simulink model "BaseEngineController_LS"  (Simulink 7.7)
settings: Solver=FixedStepDiscrete  StartTime=0.0  StopTime=10.0  RelTol=1e-3
PreLoadFcn:
  | try, eval([bdroot '_setup']); catch, eval('model_setup', ''); end
InitFcn:
  | try, eval([bdroot '_setup']); catch, eval('model_setup', ''); end
undefined symbols (not defined in the file): ECU555, High, motohawk_build_version, motohawk_trunc_name, motohawk_vardec_config_group, motohawk_vardec_path, True
libraries: MotoHawk_lib x1418, motohawk_control_primitives_lib x183, motohawk_engine_lib x32, simulink x21, motohawk_annotations_lib x9, AutoDoc_lib x8, simulink_extras x4, motohawk_ccp_examples_lib x1, motohawk_control_primitives_motoshare_lib x1
(part 13 of 27)

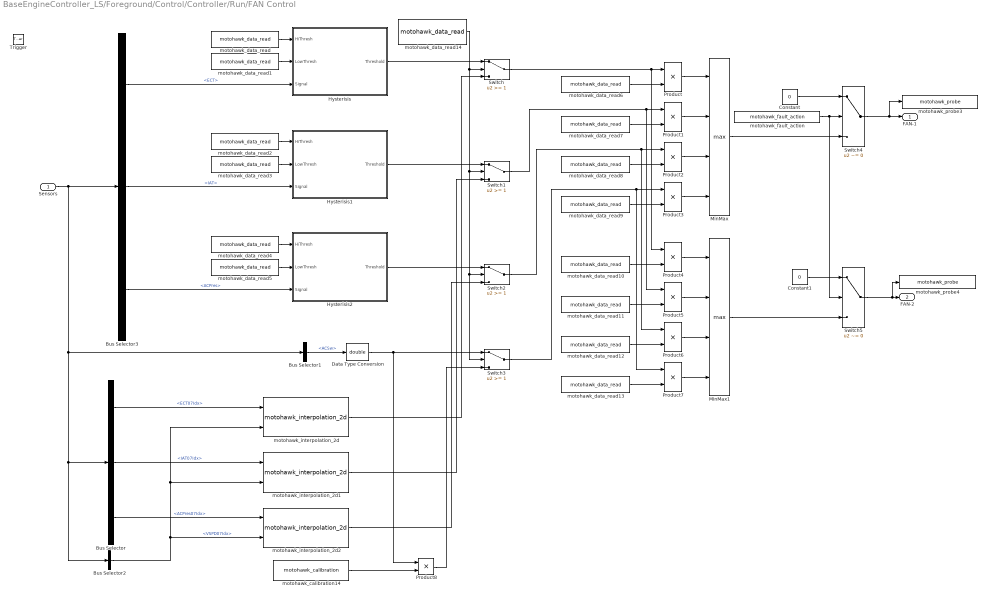
== system BaseEngineController_LS/Foreground/Control/Controller/Run/FAN Control ==
  Sensors : Inport
  Trigger : TriggerPort  TriggerType=function-call
  Bus Selector : BusSelector  OutputSignals=RawIndexes.ECT07Idx,RawIndexes.IAT07Idx,RawIndexes.ACPres07Idx
  Bus Selector1 : BusSelector  OutputSignals=Raw.Digital.ACSw
  Bus Selector2 : BusSelector  OutputSignals=RawIndexes.VSPD07Idx
  Bus Selector3 : BusSelector  OutputSignals=Raw.NonLinearSensors.ECT,Raw.NonLinearSensors.IAT,Raw.LinearSensors.ACPres
  Constant : Constant  Value=0
  Constant1 : Constant  Value=0
  Data Type Conversion : DataTypeConversion  OutDataTypeStr=double
  Hysterisis : Subsystem  AncestorBlock=motohawk_control_primitives_lib/Hysterisis
      mask Display:
      | patch([0 0 1 1], [0 0.075 0.075 0], [230/255 0/255 0/255])
      | patch([0 0 1 1], [0.025 0.05 0.05 0.025], [150/255 0/255 0/255])
      | patch([0 0 1 1], [0 0.025 0.025 0], [0/255 0/255 0/255])
      | 
      | disp('HYSTERISIS')
  Hysterisis1 : Subsystem  AncestorBlock=motohawk_control_primitives_lib/Hysterisis
      mask Display:
      | patch([0 0 1 1], [0 0.075 0.075 0], [230/255 0/255 0/255])
      | patch([0 0 1 1], [0.025 0.05 0.05 0.025], [150/255 0/255 0/255])
      | patch([0 0 1 1], [0 0.025 0.025 0], [0/255 0/255 0/255])
      | 
      | disp('HYSTERISIS')
  Hysterisis2 : Subsystem  AncestorBlock=motohawk_control_primitives_lib/Hysterisis
      mask Display:
      | patch([0 0 1 1], [0 0.075 0.075 0], [230/255 0/255 0/255])
      | patch([0 0 1 1], [0.025 0.05 0.05 0.025], [150/255 0/255 0/255])
      | patch([0 0 1 1], [0 0.025 0.025 0], [0/255 0/255 0/255])
      | 
      | disp('HYSTERISIS')
  MinMax : MinMax  Function=max  Inputs=4
  MinMax1 : MinMax  Function=max  Inputs=4
  Product{,1..8} (9 alike) : Product  RndMeth=Zero
  Switch{,1..3} (4 alike) : Switch  Threshold=1
  Switch4 : Switch  Criteria=u2 ~= 0
  Switch5 : Switch  Criteria=u2 ~= 0
  motohawk_calibration14 : MotoHawk_lib/Calibration & Probing Blocks/motohawk_calibration  nam='ACSwFanSpeed'  val=50  storage=Calibration  show_more=on  name_source=Use Parameter  data_type=uint8  read_level=1  write_level=1  ovr_cals=on  view_as=Number  enum_struct={'Disabled', 'Enabled'}  vector_style=Wide Row  use_help_units=on  help='Fan speed % req for AC Sw 0 to disable'  units='%'  use_header_enum=off  row_header_enum={}  col_header_enum={}  use_min_max=on  min_val=0  max_val=100  use_precision=off  precision=''  gain=1  offset=0  exp=1  use_mototune_group=off  mototune_group=motohawk_vardec_path(gcb)
  motohawk_data_read : MotoHawk_lib/Data Storage Blocks/motohawk_data_read  source=Lookup By Name  structure=Scalar  operation=Read scalar from location by index  sz_vec=4  sz_row=2  sz_col=3  typ=double  nam='ECTFanOn'  checkNull=on  struct_inst_name='MyData'  struct_nam='MyStruct'
  motohawk_data_read1 : MotoHawk_lib/Data Storage Blocks/motohawk_data_read  source=Lookup By Name  structure=Scalar  operation=Read scalar from location by index  sz_vec=4  sz_row=2  sz_col=3  typ=double  nam='ECTFanOff'  checkNull=on  struct_inst_name='MyData'  struct_nam='MyStruct'
  motohawk_data_read10 : MotoHawk_lib/Data Storage Blocks/motohawk_data_read  source=Lookup By Name  structure=Scalar  operation=Read scalar from location by index  sz_vec=4  sz_row=2  sz_col=3  typ=boolean  nam='Fan2ECT'  checkNull=on  struct_inst_name='MyData'  struct_nam='MyStruct'
  motohawk_data_read11 : MotoHawk_lib/Data Storage Blocks/motohawk_data_read  source=Lookup By Name  structure=Scalar  operation=Read scalar from location by index  sz_vec=4  sz_row=2  sz_col=3  typ=boolean  nam='Fan2IAT'  checkNull=on  struct_inst_name='MyData'  struct_nam='MyStruct'
  motohawk_data_read12 : MotoHawk_lib/Data Storage Blocks/motohawk_data_read  source=Lookup By Name  structure=Scalar  operation=Read scalar from location by index  sz_vec=4  sz_row=2  sz_col=3  typ=boolean  nam='Fan2ACPres'  checkNull=on  struct_inst_name='MyData'  struct_nam='MyStruct'
  motohawk_data_read13 : MotoHawk_lib/Data Storage Blocks/motohawk_data_read  source=Lookup By Name  structure=Scalar  operation=Read scalar from location by index  sz_vec=4  sz_row=2  sz_col=3  typ=boolean  nam='Fan2ACSw'  checkNull=on  struct_inst_name='MyData'  struct_nam='MyStruct'
  motohawk_data_read14 : MotoHawk_lib/Data Storage Blocks/motohawk_data_read  source=Lookup By Name  structure=Scalar  operation=Read scalar from location by index  sz_vec=4  sz_row=2  sz_col=3  typ=boolean  nam='FAN_Mode'  checkNull=on  struct_inst_name='MyData'  struct_nam='MyStruct'
  motohawk_data_read2 : MotoHawk_lib/Data Storage Blocks/motohawk_data_read  source=Lookup By Name  structure=Scalar  operation=Read scalar from location by index  sz_vec=4  sz_row=2  sz_col=3  typ=double  nam='IATFanOn'  checkNull=on  struct_inst_name='MyData'  struct_nam='MyStruct'
  motohawk_data_read3 : MotoHawk_lib/Data Storage Blocks/motohawk_data_read  source=Lookup By Name  structure=Scalar  operation=Read scalar from location by index  sz_vec=4  sz_row=2  sz_col=3  typ=double  nam='IATFanOff'  checkNull=on  struct_inst_name='MyData'  struct_nam='MyStruct'
  motohawk_data_read4 : MotoHawk_lib/Data Storage Blocks/motohawk_data_read  source=Lookup By Name  structure=Scalar  operation=Read scalar from location by index  sz_vec=4  sz_row=2  sz_col=3  typ=double  nam='ACPresFanOn'  checkNull=on  struct_inst_name='MyData'  struct_nam='MyStruct'
  motohawk_data_read5 : MotoHawk_lib/Data Storage Blocks/motohawk_data_read  source=Lookup By Name  structure=Scalar  operation=Read scalar from location by index  sz_vec=4  sz_row=2  sz_col=3  typ=double  nam='ACPresFanOff'  checkNull=on  struct_inst_name='MyData'  struct_nam='MyStruct'
  motohawk_data_read6 : MotoHawk_lib/Data Storage Blocks/motohawk_data_read  source=Lookup By Name  structure=Scalar  operation=Read scalar from location by index  sz_vec=4  sz_row=2  sz_col=3  typ=boolean  nam='Fan1ECT'  checkNull=on  struct_inst_name='MyData'  struct_nam='MyStruct'
  motohawk_data_read7 : MotoHawk_lib/Data Storage Blocks/motohawk_data_read  source=Lookup By Name  structure=Scalar  operation=Read scalar from location by index  sz_vec=4  sz_row=2  sz_col=3  typ=boolean  nam='Fan1IAT'  checkNull=on  struct_inst_name='MyData'  struct_nam='MyStruct'
  motohawk_data_read8 : MotoHawk_lib/Data Storage Blocks/motohawk_data_read  source=Lookup By Name  structure=Scalar  operation=Read scalar from location by index  sz_vec=4  sz_row=2  sz_col=3  typ=boolean  nam='Fan1ACPres'  checkNull=on  struct_inst_name='MyData'  struct_nam='MyStruct'
  motohawk_data_read9 : MotoHawk_lib/Data Storage Blocks/motohawk_data_read  source=Lookup By Name  structure=Scalar  operation=Read scalar from location by index  sz_vec=4  sz_row=2  sz_col=3  typ=boolean  nam='Fan1ACSw'  checkNull=on  struct_inst_name='MyData'  struct_nam='MyStruct'
  motohawk_fault_action : MotoHawk_lib/Fault Management Blocks/motohawk_fault_action  nam='DisableFanRun'  output_status=on  eval_nam=DisableFanRun
  motohawk_interpolation_2d : MotoHawk_lib/Lookup Tables/motohawk_interpolation_2d  nam='ECTFanSpeed'  table_data=ones(7)  show_more=off  data_type=Inherit from 'Table Data'  storage=NonAdaptive  read_level=1  write_level=1  ovr_cals=on  use_help=off  help=''  units=''  use_min_max=off  min_val=-inf  max_val=inf  use_precision=off  precision=''  gain=1  offset=0  exp=1  use_links=off  row_prelookup_block=''  col_prelookup_block=''  output_name=''  use_mototune_group=off  mototune_group=motohawk_vardec_path(gcb)
  motohawk_interpolation_2d1 : MotoHawk_lib/Lookup Tables/motohawk_interpolation_2d  nam='IATFanSpeed'  table_data=ones(7)  show_more=off  data_type=Inherit from 'Table Data'  storage=NonAdaptive  read_level=1  write_level=1  ovr_cals=on  use_help=off  help=''  units=''  use_min_max=off  min_val=-inf  max_val=inf  use_precision=off  precision=''  gain=1  offset=0  exp=1  use_links=off  row_prelookup_block=''  col_prelookup_block=''  output_name=''  use_mototune_group=off  mototune_group=motohawk_vardec_path(gcb)
  motohawk_interpolation_2d2 : MotoHawk_lib/Lookup Tables/motohawk_interpolation_2d  nam='ACPresFanSpeed'  table_data=ones(7)  show_more=off  data_type=Inherit from 'Table Data'  storage=NonAdaptive  read_level=1  write_level=1  ovr_cals=on  use_help=off  help=''  units=''  use_min_max=off  min_val=-inf  max_val=inf  use_precision=off  precision=''  gain=1  offset=0  exp=1  use_links=off  row_prelookup_block=''  col_prelookup_block=''  output_name=''  use_mototune_group=off  mototune_group=motohawk_vardec_path(gcb)
  motohawk_probe3 : MotoHawk_lib/Calibration & Probing Blocks/motohawk_probe  nam='Fan1Cmd'  show_more=on  name_source=Use Parameter  read_level=1  view_as=Number  enum_struct={'Disabled', 'Enabled'}  vector_style=Wide Row  use_help_units=on  help='FAN 1 final request'  units='%'  use_header_enum=off  row_header_enum={}  col_header_enum={}  use_precision=off  precision=''  gain=1  offset=0  exp=1  use_mototune_group=off  mototune_group=motohawk_vardec_path(gcb)
  motohawk_probe4 : MotoHawk_lib/Calibration & Probing Blocks/motohawk_probe  nam='Fan2Cmd'  show_more=on  name_source=Use Parameter  read_level=1  view_as=Number  enum_struct={'Disabled', 'Enabled'}  vector_style=Wide Row  use_help_units=on  help='Fan 2 final command'  units='%'  use_header_enum=off  row_header_enum={}  col_header_enum={}  use_precision=off  precision=''  gain=1  offset=0  exp=1  use_mototune_group=off  mototune_group=motohawk_vardec_path(gcb)
  FAN-1 : Outport
  FAN-2 : Outport  Port=2
  wires:
  Sensors/1 -> Bus Selector1/1, Bus Selector2/1, Bus Selector/1, Bus Selector3/1
  motohawk_data_read1/1 -> Hysterisis/2(LowThresh)
  motohawk_data_read/1 -> Hysterisis/1(HiThresh)
  motohawk_data_read2/1 -> Hysterisis1/1(HiThresh)
  motohawk_data_read3/1 -> Hysterisis1/2(LowThresh)
  motohawk_data_read4/1 -> Hysterisis2/1(HiThresh)
  Product/1 -> MinMax/1
  motohawk_data_read6/1 -> Product/2
  Product1/1 -> MinMax/2
  motohawk_data_read7/1 -> Product1/2
  Product2/1 -> MinMax/3
  motohawk_data_read8/1 -> Product2/2
  Product3/1 -> MinMax/4
  motohawk_data_read9/1 -> Product3/2
  Bus Selector1/1 -> Data Type Conversion/1  "<ACSw>"
  Product4/1 -> MinMax1/1
  motohawk_data_read10/1 -> Product4/2
  Product5/1 -> MinMax1/2
  motohawk_data_read11/1 -> Product5/2
  Product6/1 -> MinMax1/3
  motohawk_data_read12/1 -> Product6/2
  Product7/1 -> MinMax1/4
  motohawk_data_read5/1 -> Hysterisis2/2(LowThresh)
  motohawk_data_read13/1 -> Product7/2
  Data Type Conversion/1 -> Product8/1, Switch3/1
  motohawk_calibration14/1 -> Product8/2
  Hysterisis/1(Threshold) -> Switch/1
  motohawk_data_read14/1 -> Switch/2, Switch1/2, Switch2/2, Switch3/2
  Hysterisis1/1(Threshold) -> Switch1/1
  Hysterisis2/1(Threshold) -> Switch2/1
  Product8/1 -> Switch3/3
  motohawk_interpolation_2d2/1 -> Switch2/3
  motohawk_interpolation_2d1/1 -> Switch1/3
  motohawk_interpolation_2d/1 -> Switch/3
  Switch/1 -> Product/1, Product4/1
  Switch1/1 -> Product1/1, Product5/1
  Switch2/1 -> Product2/1, Product6/1
  Switch3/1 -> Product3/1, Product7/1
  Switch4/1 -> FAN-1/1, motohawk_probe3/1
  MinMax/1 -> Switch4/3
  motohawk_fault_action/1 -> Switch4/2, Switch5/2
  Constant/1 -> Switch4/1
  MinMax1/1 -> Switch5/3
  Switch5/1 -> FAN-2/1, motohawk_probe4/1
  Constant1/1 -> Switch5/1
  Bus Selector/1 -> motohawk_interpolation_2d/1  "<ECT07Idx>"
  Bus Selector/2 -> motohawk_interpolation_2d1/1  "<IAT07Idx>"
  Bus Selector/3 -> motohawk_interpolation_2d2/1  "<ACPres07Idx>"
  Bus Selector2/1 -> motohawk_interpolation_2d2/2, motohawk_interpolation_2d1/2, motohawk_interpolation_2d/2  "<VSPD07Idx>"
  Bus Selector3/1 -> Hysterisis/3(Signal)  "<ECT>"
  Bus Selector3/2 -> Hysterisis1/3(Signal)  "<IAT>"
  Bus Selector3/3 -> Hysterisis2/3(Signal)  "<ACPres>"

== system BaseEngineController_LS/Foreground/Control/Controller/Run/Fuel System Manager ==
  Sensors : Inport
  O2_Info : Inport  Port=2
  Bus Selector : BusSelector  OutputSignals=O2Error.O2Cals
  DesiredFuelCalc : Subsystem
  Fuel Calculation : Subsystem
      mask Display:
      | patch([0 0 1 1], 0.5*[0 0.075 0.075 0], [230/255 0/255 0/255])
      | patch([0 0 1 1], 0.5*[0.025 0.05 0.05 0.025], [150/255 0/255 0/255])
      | patch([0 0 1 1], 0.5*[0 0.025 0.025 0], [0/255 0/255 0/255])
      | 
      | disp('BASE FUEL');
  Injector Manager : Subsystem  TreatAsAtomicUnit=on
      mask Display:
      | patch([0 0 1 1], 0.5*[0 0.075 0.075 0], [230/255 0/255 0/255])
      | patch([0 0 1 1], 0.5*[0.025 0.05 0.05 0.025], [150/255 0/255 0/255])
      | patch([0 0 1 1], 0.5*[0 0.025 0.025 0], [0/255 0/255 0/255])
  O2 Fuel Adapt : Subsystem  TreatAsAtomicUnit=on
      mask Display:
      | patch([0 0 1 1], 0.5*[0 0.075 0.075 0], [230/255 0/255 0/255])
      | patch([0 0 1 1], 0.5*[0.025 0.05 0.05 0.025], [150/255 0/255 0/255])
      | patch([0 0 1 1], 0.5*[0 0.025 0.025 0], [0/255 0/255 0/255])
  DesiredFuel : Outport
  InjTiming : Outport  Port=2
  EOI : Outport  Port=3
  wires:
  O2_Info/1 -> Fuel Calculation/2(O2Info), O2 Fuel Adapt/1(O2 Info), Bus Selector/1
  Fuel Calculation/1(Fuel) -> Injector Manager/1(Fuel)
  Injector Manager/1(PrimaryInjTiming) -> InjTiming/1
  Injector Manager/2(MakeUpInjTiming) -> EOI/1
  Sensors/1 -> O2 Fuel Adapt/2(Sensors), Injector Manager/2(Sensors), Fuel Calculation/1(Sensors)
  DesiredFuelCalc/1(DesiredFuel) -> DesiredFuel/1
  Bus Selector/1 -> DesiredFuelCalc/2(BankCals)  "<O2Cals>"
  Injector Manager/3(FPC) -> DesiredFuelCalc/1(FPC)
  O2 Fuel Adapt/1("Adapt Fuel Mult Bank A ") -> DesiredFuelCalc/3(BankAMult)
  O2 Fuel Adapt/2(Adapt Fuel Mult Bank B) -> DesiredFuelCalc/4(BankBMult)

== system BaseEngineController_LS/Foreground/Control/Controller/Run/IAC Characterization ==
  MinGovINFO : Inport
  Bus Selector4 : BusSelector  OutputSignals=OnIdle,BaseAirOfst,MinGovAirPID
  Constant : Constant  Value=0
  Constant1 : Constant  Value=100
  Constant2 : Constant  Value=0
  Logical Operator : Logic  Operator=NOT  AllPortsSameDT=off  OutDataTypeStr=boolean
  Sum : Sum  Inputs=|+-
  Sum2 : Sum
  Switch1 : Switch  Criteria=u2 > Threshold
  Switch4 : Switch  Threshold=1
  motohawk_data_read : MotoHawk_lib/Data Storage Blocks/motohawk_data_read  source=Lookup By Name  structure=Scalar  operation=Read scalar from location by index  sz_vec=4  sz_row=2  sz_col=3  typ=uint8  nam='IACType'  checkNull=on  struct_inst_name='MyData'  struct_nam='MyStruct'
  IAC-P : Outport
  IAC-S : Outport  Port=2
  wires:
  motohawk_data_read/1 -> Switch1/2
  Switch1/1 -> IAC-S/1
  Constant/1 -> Switch1/3
  Constant1/1 -> Sum/1
  Sum/1 -> Switch1/1
  Logical Operator/1 -> Switch4/2
  Bus Selector4/1 -> Logical Operator/1  "<OnIdle>"
  Bus Selector4/3 -> Sum2/2  "<MinGovAirPID>"
  Bus Selector4/2 -> Sum2/1  "<BaseAirOfst>"
  MinGovINFO/1 -> Bus Selector4/1
  Switch4/1 -> Sum/2, IAC-P/1
  Constant2/1 -> Switch4/1
  Sum2/1 -> Switch4/3

== system BaseEngineController_LS/Foreground/Control/Controller/Run/MaxGovernor ==
  MinGovInfo : Inport
  Sensors : Inport  Port=2
  Trigger : TriggerPort  TriggerType=function-call
  Bus Creator : BusCreator  Inputs=2
  Bus Selector1 : BusSelector  OutputSignals=BaseAirOfst
  Bus Selector2 : BusSelector  OutputSignals=RawProcessed.ETCRequest
  Bus Selector3 : BusSelector  OutputSignals=VirtualIndexes.RPMAccel17Idx
  Bus Selector4 : BusSelector  OutputSignals=Raw.RPMInst
  Bus Selector5 : BusSelector  OutputSignals=Raw.RPMInst,Raw.Digital.ClutchSw
  Data Type Conversion : DataTypeConversion  OutDataTypeStr=double
  Data Type Conversion1 : DataTypeConversion  OutDataTypeStr=double
  I-Term Preload : Subsystem  TreatAsAtomicUnit=on
  MaxGovState : Subsystem
  Ramp RPM : Subsystem
      mask Display: disp('RAMP RPM\nINTO STEADY-STATE');
  Sum : Sum  Inputs=|++
  Terminator : Terminator
  Trigger Pre-load : Subsystem
  Unit Delay : UnitDelay  SampleTime=-1
  Universal PID (Tunable & Scheduled) : Subsystem  AncestorBlock=motohawk_control_primitives_lib/Universal PID (Tunable & Scheduled)  mask(Universal PID (Tunable)){nam='MaxGov', prefix='MaxGov', samp_time=-1, units='%', group=motohawk_vardec_path(gcb)}
      mask prompts: nam "Name"; samp_time "Sample Time"; group "MotoTune Group String"
      mask help:
      | This block wraps a 'Universal PID' block to provide gain scheduling and calibrations and probes for most parameters.
      |
      | If 'Sample Time' is -1, then extra code and RAM will be generated to dynamically calculate dt.
      mask init:
      | grp = [group ' | ' nam];
      mask Display:
      | patch([0 0 1 1], [0 0.075 0.075 0], [230/255 0/255 0/255])
      | patch([0 0 1 1], [0.025 0.05 0.05 0.025], [150/255 0/255 0/255])
      | patch([0 0 1 1], [0 0.025 0.025 0], [0/255 0/255 0/255])
      | 
      | disp([nam '\n(PID w/ Gain Schedules)']);
  motohawk_probe : MotoHawk_lib/Calibration & Probing Blocks/motohawk_probe  nam='TPSRequestLookupAirOfst'  show_more=on  name_source=Use Parameter  read_level=1  view_as=Number  enum_struct={'Disabled', 'Enabled'}  vector_style=Wide Row  use_help_units=on  help=''  units=''  use_header_enum=off  row_header_enum={}  col_header_enum={}  use_precision=on  precision=''  gain=1  offset=0  exp=1  use_mototune_group=on  mototune_group=motohawk_vardec_path(gcb)
  motohawk_probe2 : MotoHawk_lib/Calibration & Probing Blocks/motohawk_probe  nam='MaxGovOutput'  show_more=on  name_source=Use Parameter  read_level=1  view_as=Number  enum_struct={'Disabled', 'Enabled'}  vector_style=Wide Row  use_help_units=on  help=''  units=''  use_header_enum=off  row_header_enum={}  col_header_enum={}  use_precision=on  precision=''  gain=1  offset=0  exp=1  use_mototune_group=on  mototune_group=motohawk_vardec_path(gcb)
  MaxGovInfo : Outport
  wires:
  MinGovInfo/1 -> Bus Selector1/1
  Bus Creator/1 -> MaxGovInfo/1
  Bus Selector1/1 -> Sum/1  "<BaseAirOfst>"
  Bus Selector2/1 -> Sum/2  "<ETCRequest>"
  Sensors/1 -> Bus Selector2/1, Bus Selector5/1, Bus Selector3/1, Bus Selector4/1, MaxGovState/3(Sensors)
  Sum/1 -> I-Term Preload/1(TotalETCReq), MaxGovState/2(TotalETCReq), motohawk_probe/1
  Bus Selector3/1 -> I-Term Preload/2(RPMAccelIdx)  "<RPMAccel17Idx>"
  I-Term Preload/1(ITerm Preload) -> Universal PID (Tunable & Scheduled)/1(ITerm IC)
  MaxGovState/1(ETCMode) -> Bus Creator/1, Unit Delay/1  "MaxGovState"
  Trigger Pre-load/1(Trigger) -> MaxGovState/1(RPMEntryCriteria)
  Bus Selector4/1 -> Data Type Conversion1/1  "<RPMInst>"
  Bus Selector5/1 -> Trigger Pre-load/1(RPM)  "<RPMInst>"
  Universal PID (Tunable & Scheduled)/1(MaxGovOut) -> Bus Creator/2, motohawk_probe2/1  "MaxGovPID"
  Universal PID (Tunable & Scheduled)/2(MaxGovITerm) -> Terminator/1
  Trigger Pre-load/2(BaseRPMSetpoint) -> Data Type Conversion/1
  Unit Delay/1 -> Ramp RPM/1(OnIdle)
  MaxGovState/3(PIDHold) -> Universal PID (Tunable & Scheduled)/3(Hold PID)
  Ramp RPM/1(RPMSetPt) -> Universal PID (Tunable & Scheduled)/4(SetPoint)
  MaxGovState/2(PIDReset) -> Universal PID (Tunable & Scheduled)/2(Reset All)
  Bus Selector5/2 -> Trigger Pre-load/2(GearState)  "<ClutchSw>"
  Data Type Conversion/1 -> Ramp RPM/2(TargetRPM), MaxGovState/4(TargetRPM)
  Data Type Conversion1/1 -> Universal PID (Tunable & Scheduled)/5(Actual), Ramp RPM/3(RPM)

== system BaseEngineController_LS/Foreground/Control/Controller/Run/MinGovernor ==
  Sensors : Inport
  AC : Inport  Port=2
  Trigger : TriggerPort  TriggerType=function-call
  AiflowOffset : Subsystem  TreatAsAtomicUnit=on
  Base Airflow Table Adapt : Subsystem  TreatAsAtomicUnit=on
  Base RPM Set Pt : Subsystem  TreatAsAtomicUnit=on
  Bus Creator2 : BusCreator  Inputs=5
  Bus Selector : BusSelector  OutputSignals=Raw.RPM
  Bus Selector1 : BusSelector  OutputSignals=Raw.RPMInst
  Constant1 : Constant  Value=0  OutDataTypeStr=Inherit: Inherit via back propagation  SampleTime=-1
  Data Type Conversion : DataTypeConversion  OutDataTypeStr=double
  Data Type Conversion1 : DataTypeConversion  SaturateOnIntegerOverflow=on  RndMeth=Zero
  Handoff Alpha : motohawk_control_primitives_lib/Handoff Alpha  SystemSampleTime=-1  samp_time=-1
  Hit  Crossing1 : HitCross  HitCrossingOffset=.5  HitCrossingDirection=falling
  Idle State Determination : Subsystem
      mask Display: disp('IDLE STATE\nDETERMINATION');
  Logical Operator : Logic  Operator=OR  AllPortsSameDT=off
  MotoringDetection : Subsystem
  OnIdle State : motohawk_control_primitives_lib/CompareTo  SystemSampleTime=-1  op===  val=0
  Product : Product  SaturateOnIntegerOverflow=on  InputSameDT=on  OutDataTypeStr=Inherit: Same as first input
  Product1 : Product  SaturateOnIntegerOverflow=on  InputSameDT=on  OutDataTypeStr=Inherit: Same as first input
  Ramp RPM : Subsystem
      mask Display: disp('RAMP RPM\nINTO IDLE STATE');
  Unit Delay1 : UnitDelay  SampleTime=-1
  Unit Delay2 : UnitDelay  SampleTime=-1
  Unit Delay3 : UnitDelay  SampleTime=-1
  Universal PD (Tunable & Scheduled) : Subsystem  AncestorBlock=motohawk_control_primitives_lib/Universal PD (Tunable & Scheduled)  mask(Universal PD (Tunable)){nam='SpkMinGov', prefix='SpkMinGov', samp_time=-1, units='degCA', group=motohawk_vardec_path(gcb)}
      mask prompts: nam "Name"; samp_time "Sample Time"; group "MotoTune Group String"
      mask help:
      | This block wraps a 'Universal PD' block to provide gain scheduling and calibrations and probes for most parameters.
      |
      | If 'Sample Time' is -1, then extra code and RAM will be generated to dynamically calculate dt.
      mask init:
      | grp = [group ' | ' nam];
      mask Display:
      | patch([0 0 1 1], [0 0.075 0.075 0], [230/255 0/255 0/255])
      | patch([0 0 1 1], [0.025 0.05 0.05 0.025], [150/255 0/255 0/255])
      | patch([0 0 1 1], [0 0.025 0.025 0], [0/255 0/255 0/255])
      | 
      | disp([nam '\n(PD w/ Gain Schedules)']);
  Universal PID (Tunable & Scheduled) : Subsystem  AncestorBlock=motohawk_control_primitives_lib/Universal PID (Tunable & Scheduled)  mask(Universal PID (Tunable)){nam='AirMinGov', prefix='AirMinGov', samp_time=-1, units='%', group=motohawk_vardec_path(gcb)}
      mask prompts: nam "Name"; samp_time "Sample Time"; group "MotoTune Group String"
      mask help:
      | This block wraps a 'Universal PID' block to provide gain scheduling and calibrations and probes for most parameters.
      |
      | If 'Sample Time' is -1, then extra code and RAM will be generated to dynamically calculate dt.
      mask init:
      | grp = [group ' | ' nam];
      mask Display:
      | patch([0 0 1 1], [0 0.075 0.075 0], [230/255 0/255 0/255])
      | patch([0 0 1 1], [0.025 0.05 0.05 0.025], [150/255 0/255 0/255])
      | patch([0 0 1 1], [0 0.025 0.025 0], [0/255 0/255 0/255])
      | 
      | disp([nam '\n(PID w/ Gain Schedules)']);
  motohawk_calibration3 : MotoHawk_lib/Calibration & Probing Blocks/motohawk_calibration  nam='IdleExitTimeConst'  val=0.005  storage=Calibration  show_more=on  name_source=Use Parameter  data_type=Inherit from 'Default Value'  read_level=1  write_level=1  ovr_cals=on  view_as=Number  enum_struct={'Disabled', 'Enabled'}  vector_style=Wide Row  use_help_units=on  help='Time constant for idle air and spark ramp out'  units='sec'  use_header_enum=off  row_header_enum={}  col_header_enum={}  use_min_max=off  min_val=0  max_val=100  use_precision=on  precision='2.3'  gain=1  offset=0  exp=1  use_mototune_group=on  mototune_group=motohawk_vardec_path(gcb)
  motohawk_probe2 : MotoHawk_lib/Calibration & Probing Blocks/motohawk_probe  nam='IdleHandOffMult'  show_more=on  name_source=Use Parameter  read_level=1  view_as=Number  enum_struct={'Disabled', 'Enabled'}  vector_style=Wide Row  use_help_units=off  help=''  units=''  use_header_enum=off  row_header_enum={}  col_header_enum={}  use_precision=off  precision=''  gain=1  offset=0  exp=1  use_mototune_group=on  mototune_group=motohawk_vardec_path(gcb)
  motohawk_probe3 : MotoHawk_lib/Calibration & Probing Blocks/motohawk_probe  nam='MinGovReset'  show_more=on  name_source=Use Parameter  read_level=1  view_as=Number  enum_struct={'Disabled', 'Enabled'}  vector_style=Wide Row  use_help_units=on  help=''  units=''  use_header_enum=off  row_header_enum={}  col_header_enum={}  use_precision=on  precision=''  gain=1  offset=0  exp=1  use_mototune_group=on  mototune_group=motohawk_vardec_path(gcb)
  motohawk_probe4 : MotoHawk_lib/Calibration & Probing Blocks/motohawk_probe  nam='AirMinGovOutput'  show_more=on  name_source=Use Parameter  read_level=1  view_as=Number  enum_struct={'Disabled', 'Enabled'}  vector_style=Wide Row  use_help_units=on  help='Total output from min. gov. air PID controller.'  units='%'  use_header_enum=off  row_header_enum={}  col_header_enum={}  use_precision=on  precision=''  gain=1  offset=0  exp=1  use_mototune_group=on  mototune_group=motohawk_vardec_path(gcb)
  motohawk_probe5 : MotoHawk_lib/Calibration & Probing Blocks/motohawk_probe  nam='SpkMinGovOutput'  show_more=on  name_source=Use Parameter  read_level=1  view_as=Number  enum_struct={'Disabled', 'Enabled'}  vector_style=Wide Row  use_help_units=on  help=''  units=''  use_header_enum=off  row_header_enum={}  col_header_enum={}  use_precision=on  precision=''  gain=1  offset=0  exp=1  use_mototune_group=on  mototune_group=motohawk_vardec_path(gcb)
  MinGovInfo : Outport
  wires:
  Sensors/1 -> Bus Selector1/1, Bus Selector/1, Base RPM Set Pt/1(Sensors), Idle State Determination/1(Sensors), AiflowOffset/1(Sensors)
  Bus Selector/1 -> Universal PD (Tunable & Scheduled)/1(Actual), Universal PID (Tunable & Scheduled)/1(Actual), MotoringDetection/1(ActualRPM)  "<RPM>"
  Idle State Determination/1(OnIdle) -> Bus Creator2/2, Ramp RPM/1(OnIdle), Base Airflow Table Adapt/Enable, Base Airflow Table Adapt/1(Idle State), Handoff Alpha/1  "OnIdle"
  Ramp RPM/1(RPMSetPt) -> Bus Creator2/3, Universal PD (Tunable & Scheduled)/2(SetPoint), Universal PID (Tunable & Scheduled)/2(SetPoint), MotoringDetection/2(SetpointRPM)  "MinGovSetpoint"
  Base RPM Set Pt/1(RPMSetPt) -> Idle State Determination/3(TargetRPM), Data Type Conversion/1
  AiflowOffset/1(BaseAirOffset) -> Bus Creator2/1  "BaseAirOfst"
  Bus Selector1/1 -> Ramp RPM/3(RPM)  "<RPMInst>"
  MotoringDetection/1(MotoringFlag) -> Unit Delay2/1
  Unit Delay2/1 -> Hit  Crossing1/1
  Hit  Crossing1/1 -> Data Type Conversion1/1
  Universal PID (Tunable & Scheduled)/2(MinGovITerm) -> Unit Delay1/1
  Handoff Alpha/1 -> motohawk_probe2/1, Product/1, Product1/1, OnIdle State/1
  motohawk_calibration3/1 -> Handoff Alpha/3
  Constant1/1 -> Handoff Alpha/2
  Data Type Conversion1/1 -> Logical Operator/2
  Logical Operator/1 -> Universal PID (Tunable & Scheduled)/3(ResetAll), motohawk_probe3/1
  OnIdle State/1 -> Universal PD (Tunable & Scheduled)/3(ResetAll), Logical Operator/1
  Universal PD (Tunable & Scheduled)/1(SpkOut) -> Product/2
  Universal PID (Tunable & Scheduled)/1(MinGovOut) -> Product1/2
  Product1/1 -> Bus Creator2/5, Unit Delay3/1, motohawk_probe4/1  "MinGovAirPID"
  Unit Delay1/1 -> Base Airflow Table Adapt/2(ITerm)
  Unit Delay3/1 -> Idle State Determination/2(MinGovOutput)
  Bus Creator2/1 -> MinGovInfo/1  "MinGovInfo"
  AC/1 -> AiflowOffset/2(AC)
  Data Type Conversion/1 -> Ramp RPM/2(TargetRPM)
  Product/1 -> Bus Creator2/4, motohawk_probe5/1  "IdleSpk"

== system BaseEngineController_LS/Foreground/Control/Controller/Run/O2 Control ==
  Reset : Inport
  Sensors : Inport  Port=2
  Desired_Equiv : Inport  Port=3
  Bus Creator : BusCreator
  Bus Creator1 : BusCreator  Inputs=3
  Bus Creator2 : BusCreator  Inputs=1
  Bus Selector1 : BusSelector  OutputSignals=DesEquivRatio
  Bus Selector2 : BusSelector  OutputSignals=RawProcessed.O2Delagged.O2BankADelagged
  Bus Selector3 : BusSelector  OutputSignals=Raw.CAN.O2_BUS.BANK1.DataValidState,Raw.CAN.O2_BUS.BANK2.DataValidState
  Bus Selector4 : BusSelector  OutputSignals=SSEng,VirtualIndexes.ECTKeyUp09Idx,RawProcessed.TimeSinceRun
  Bus Selector5 : BusSelector  OutputSignals=RawProcessed.O2Delagged.O2BankBDelagged
  Logical Operator : Logic  Operator=NOT  AllPortsSameDT=off  OutDataTypeStr=boolean
  Logical Operator1 : Logic  Operator=NOT  AllPortsSameDT=off  OutDataTypeStr=boolean
  Map O2 Sensors to V8 Cylinders : Subsystem  AncestorBlock=motohawk_engine_lib/Closed-Loop O2 Control - Dual Bank/Map O2 Sensors to V8 Cylinders
      mask Display: disp('');
  O2 Control State Determination : Subsystem
  O2 PID Calibrations : Subsystem
  O2 PID Controller Bank A : Subsystem  AncestorBlock=motohawk_engine_lib/O2A  TreatAsAtomicUnit=on  mask(Closed-Loop O2 Control){display_group='Engine Control | Run | Fuel | O2 Control', cal_group=motohawk_vardec_path(gcb)}
      mask prompts: display_group "MotoTune Display Group"; cal_group "MotoTune Calibration Group"
      mask Display:
      | patch([0 0 1 1], 0.5*[0 0.075 0.075 0], [230/255 0/255 0/255])
      | patch([0 0 1 1], 0.5*[0.025 0.05 0.05 0.025], [150/255 0/255 0/255])
      | patch([0 0 1 1], 0.5*[0 0.025 0.025 0], [0/255 0/255 0/255])
      | 
      | disp('Liquid O2 Control');
  O2 PID Controller Bank B : Subsystem  AncestorBlock=motohawk_engine_lib/O2A  TreatAsAtomicUnit=on  mask(Closed-Loop O2 Control){display_group='Engine Control | Run | Fuel | O2 Control', cal_group=motohawk_vardec_path(gcb)}
      mask prompts: display_group "MotoTune Display Group"; cal_group "MotoTune Calibration Group"
      mask Display:
      | patch([0 0 1 1], 0.5*[0 0.075 0.075 0], [230/255 0/255 0/255])
      | patch([0 0 1 1], 0.5*[0.025 0.05 0.05 0.025], [150/255 0/255 0/255])
      | patch([0 0 1 1], 0.5*[0 0.025 0.025 0], [0/255 0/255 0/255])
      | 
      | disp('Liquid O2 Control');
  O2Arb : Subsystem
  O2Disable : Subsystem
  motohawk_data_def : MotoHawk_lib/Data Storage Blocks/motohawk_data_def  nam='DisableO2FaultAction'  container_nam=''  data=0  typ=boolean  struct_nam='MyStruct'  storage=Volatile  outputRef=off  use_vardec=off  window=Calibration  read_level=1  write_level=1  ovr_cals=on  view_as=Number  enum_struct={'Disabled', 'Enabled'}  vector_style=Wide Row  use_help_units=on  help=''  units=''  use_header_enum=off  row_header_enum=''  col_header_enum=''  use_min_max=off  min_val=-inf  max_val=inf  use_precision=off  precision=''  gain=1  offset=0  exp=1  use_mototune_group=off  mototune_group=motohawk_vardec_path(gcb)  eval_name=DisableO2FaultAction  data_stores=motohawk_sfun_data_def_data_stores  struct_instances=motohawk_sfun_data_def_struct_instances  vardecs=motohawk_sfun_data_def_vardecs
  motohawk_data_write : MotoHawk_lib/Data Storage Blocks/motohawk_data_write  source=Lookup By Name  structure=Scalar  operation=Write scalar into location by index  sz_vec=-1  sz_row=3  sz_col=2  typ=boolean  nam='DisableO2FaultAction'  checkNull=on  write_read_only=off  struct_inst_name='Struct1'  struct_name='MyStruct'
  O2_Info : Outport
  wires:
  Logical Operator1/1 -> O2 PID Controller Bank A/5(Reset), O2 PID Controller Bank B/5(Reset)
  Logical Operator/1 -> O2 PID Controller Bank A/1(Hold PID), O2 PID Controller Bank B/1(Hold PID)
  Reset/1 -> Logical Operator1/1
  Bus Creator1/1 -> Bus Creator/4  "O2Error"
  Desired_Equiv/1 -> Bus Creator/1, Bus Selector1/1  "DesiredLambda"
  Sensors/1 -> Bus Selector4/1, Bus Selector3/1, Bus Selector2/1, O2 PID Calibrations/1(Sensors), Bus Selector5/1
  O2 Control State Determination/1(O2Control) -> Bus Creator2/1, Logical Operator/1, O2Arb/1(BankEnable)  "BankAEnable"
  Bus Creator2/1 -> Bus Creator/2  "O2ControlEnable"
  O2 PID Calibrations/1(Calibrations) -> O2 PID Controller Bank A/4(Calibrations), O2 PID Controller Bank B/4(Calibrations)
  Bus Selector1/1 -> O2 Control State Determination/5(DesEquivRatio), O2 PID Controller Bank A/3(DesEquivRatio), O2 PID Controller Bank B/3(DesEquivRatio)  "<DesEquivRatio>"
  Bus Selector2/1 -> O2 PID Controller Bank A/2(O2Sensor)  "<O2BankADelagged>"
  Bus Selector4/1 -> O2 Control State Determination/2(SSEngOpr)  "<SSEng>"
  Bus Selector4/2 -> O2 Control State Determination/3(ECT_KeyUp_Idx)  "<ECTKeyUp09Idx>"
  Bus Selector4/3 -> O2 Control State Determination/4(TimeSinceRun)  "<TimeSinceRun>"
  Bus Creator/1 -> O2_Info/1  "O2Info"
  Bus Selector3/1 -> O2Disable/1(Bank1Valid)  "<DataValidState>"
  Bus Selector3/2 -> O2Disable/2(Bank2Valid)  "<DataValidState>"
  O2Disable/1(Out1) -> motohawk_data_write/1, O2 Control State Determination/1(O2 Sensor Fault)
  O2Arb/1(FuelMult) -> Bus Creator/3
  Map O2 Sensors to V8 Cylinders/1(O2FuelMult [per-cylinder]) -> O2Arb/2(O2PidOut)
  O2 PID Controller Bank A/1(FuelMult) -> Map O2 Sensors to V8 Cylinders/1(O2FuelMultA)  "O2FuelMult"
  O2 PID Controller Bank B/1(FuelMult) -> Map O2 Sensors to V8 Cylinders/2(O2FuelMultB)
  Bus Selector5/1 -> O2 PID Controller Bank B/2(O2Sensor)  "<O2BankBDelagged>"
  O2 PID Controller Bank A/2(O2 Error) -> Bus Creator1/2  "O2ITerm_BankA"
  Map O2 Sensors to V8 Cylinders/2(BankCylSelectCal) -> Bus Creator1/1  "O2Cals"
  O2 PID Controller Bank B/2(O2 Error) -> Bus Creator1/3  "O2ITerm_BankB"

== system BaseEngineController_LS/Foreground/Control/Controller/Run/Spark Manager ==
  DesEquivRatio : Inport
  Sensors : Inport  Port=2
  RPM_Ctrl_Ofst : Inport  Port=3
  DFCOInfo : Inport  Port=4
  Trigger : TriggerPort  TriggerType=function-call
  Apply Offsets to Base Spark Advance1 : Sum  Inputs=+++  SaturateOnIntegerOverflow=on  InputSameDT=on
  Apply Offsets to Base Spark Advance3 : Sum  Inputs=++++  SaturateOnIntegerOverflow=on  InputSameDT=on
  Bus Selector : BusSelector  OutputSignals=RawIndexes.MAP09Idx,RawIndexes.RPM09Idx
  Bus Selector1 : BusSelector  OutputSignals=RawIndexes.MAP17Idx,RawIndexes.RPM17Idx
  Bus Selector2 : BusSelector  OutputSignals=IdleSpk
  Bus Selector3 : BusSelector  OutputSignals=SpkOut
  Bus Selector4 : BusSelector  OutputSignals=OnIdle
  Bus Selector5 : BusSelector  OutputSignals=DesEquivRatio
  Desired Eq Ratio Offset : Subsystem
  Ethanol Spark Offset : Subsystem
  Spark Advance Rate Limiter : Subsystem
  SparkAdvanceLimiter : Subsystem
  Temp Comp Offset : Subsystem
  motohawk_interpolation_2d1 : MotoHawk_lib/Lookup Tables/motohawk_interpolation_2d  nam='BaseSparkEnergy'  table_data=ones(9)  show_more=on  data_type=Inherit from 'Table Data'  storage=NonAdaptive  read_level=1  write_level=1  ovr_cals=on  use_help=on  help='Spark energy - Run state'  units='mJ'  use_min_max=off  min_val=-inf  max_val=inf  use_precision=on  precision=''  gain=1  offset=0  exp=1  use_links=off  row_prelookup_block=''  col_prelookup_block=''  output_name=''  use_mototune_group=on  mototune_group=motohawk_vardec_path(gcb)
  motohawk_interpolation_2d2 : MotoHawk_lib/Lookup Tables/motohawk_interpolation_2d  nam='SparkAdv'  table_data=ones(17)*10  show_more=on  data_type=Inherit from 'Table Data'  storage=NonAdaptive  read_level=1  write_level=1  ovr_cals=on  use_help=on  help='Base spark advance map.'  units='degBTDC'  use_min_max=on  min_val=-inf  max_val=inf  use_precision=on  precision=''  gain=1  offset=0  exp=1  use_links=off  row_prelookup_block=''  col_prelookup_block=''  output_name=''  use_mototune_group=on  mototune_group=motohawk_vardec_path(gcb)
  motohawk_probe : MotoHawk_lib/Calibration & Probing Blocks/motohawk_probe  nam='Spark_Adv_Prb'  show_more=off  name_source=Use Parameter  read_level=1  view_as=Number  enum_struct={'Disabled', 'Enabled'}  vector_style=Wide Row  use_help_units=off  help=''  units=''  use_header_enum=off  row_header_enum={}  col_header_enum={}  use_precision=off  precision=''  gain=1  offset=0  exp=1  use_mototune_group=off  mototune_group=motohawk_vardec_path(gcb)
  SparkEnergy : Outport
  SpkAdv : Outport  Port=2
  wires:
  SparkAdvanceLimiter/1(SparkAdv) -> Spark Advance Rate Limiter/1(DesSparkAdv), motohawk_probe/1
  Sensors/1 -> Bus Selector/1, Bus Selector1/1, Temp Comp Offset/1(Sensors), Ethanol Spark Offset/1(Sensors), SparkAdvanceLimiter/3(Sensors), Desired Eq Ratio Offset/1(Sensors)
  Bus Selector4/1 -> SparkAdvanceLimiter/2(OnIdle)  "<OnIdle>"
  Apply Offsets to Base Spark Advance1/1 -> SparkAdvanceLimiter/1(DesSparkAdv)
  Spark Advance Rate Limiter/1(SparkAdv) -> SpkAdv/1
  Bus Selector/1 -> motohawk_interpolation_2d1/1  "<MAP09Idx>"
  Bus Selector/2 -> motohawk_interpolation_2d1/2  "<RPM09Idx>"
  Bus Selector1/1 -> motohawk_interpolation_2d2/1  "<MAP17Idx>"
  Bus Selector1/2 -> motohawk_interpolation_2d2/2  "<RPM17Idx>"
  Temp Comp Offset/1(TempSpkOfst) -> Apply Offsets to Base Spark Advance3/2
  Apply Offsets to Base Spark Advance3/1 -> Apply Offsets to Base Spark Advance1/1
  RPM_Ctrl_Ofst/1 -> Bus Selector2/1, Bus Selector4/1
  Bus Selector2/1 -> Apply Offsets to Base Spark Advance1/2  "<IdleSpk>"
  motohawk_interpolation_2d1/1 -> SparkEnergy/1
  motohawk_interpolation_2d2/1 -> Apply Offsets to Base Spark Advance3/1  "RichEquivRatioTargetDelta"
  Ethanol Spark Offset/1(EthanolSpkOfst) -> Apply Offsets to Base Spark Advance3/3
  DFCOInfo/1 -> Bus Selector3/1
  Bus Selector3/1 -> Apply Offsets to Base Spark Advance1/3  "<SpkOut>"
  DesEquivRatio/1 -> Bus Selector5/1
  Bus Selector5/1 -> Desired Eq Ratio Offset/2(DesiredEqRatio)  "<DesEquivRatio>"
  Desired Eq Ratio Offset/1(EqRatioSpkOfst) -> Apply Offsets to Base Spark Advance3/4
